simulink model "envelope_detector"  (R2021a)
settings: Solver=VariableStepAuto  StartTime=0.0  StopTime=10.0  RelTol=1e-3
libraries: dsparch4 x1, dspsigops x1
settings Model: Creator=Fatiha  LastModifiedBy=Fatiha

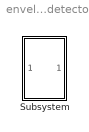
== system envelope_detector ==
  Subsystem : Subsystem

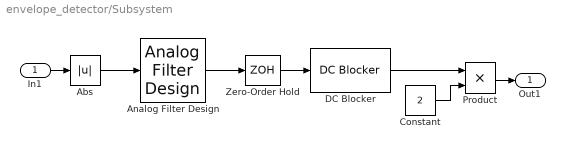
== system envelope_detector/Subsystem ==
  In1 : Inport
  Abs : Abs
  Analog Filter Design : dsparch4/Analog Filter Design  method=Butterworth  filttype=Lowpass  N=8  Wlo=2*pi*0.5e3  Whi=80  Rp=2  Rs=40
  Constant : Constant  Value=2
  DC Blocker : dspsigops/DC Blocker  Algorithm=IIR  NormalizedBandwidth=0.001  Length=8  Order=6  SimulateUsing=Code generation
      settings: SourceProductBaseCode=DS
  Product : Product
  Zero-Order Hold : ZeroOrderHold  SampleTime=-1
  Out1 : Outport
  wires:
  DC Blocker/1 -> Product/1
  Product/1 -> Out1/1
  In1/1 -> Abs/1
  Constant/1 -> Product/2
  Analog Filter Design/1 -> Zero-Order Hold/1
  Zero-Order Hold/1 -> DC Blocker/1
  Abs/1 -> Analog Filter Design/1
